simulink model "eeg_sim"  (R2025b)
settings: Solver=VariableStepAuto  StartTime=0.0  StopTime=10000  RelTol=1e-3
libraries: dspnetwork x1
settings Model: Creator=rashe  LastModifiedBy=rashe

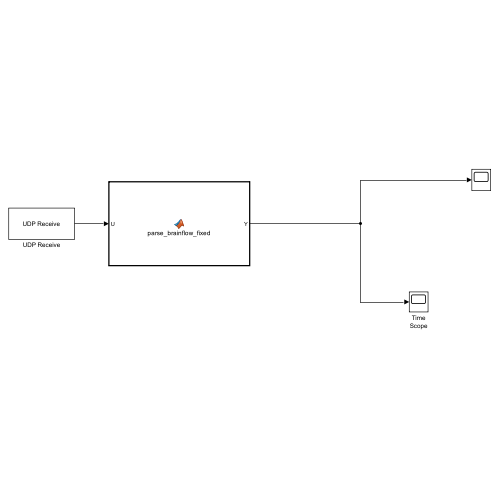
[thumbnail: Simulink's stored preview of the top-level diagram]
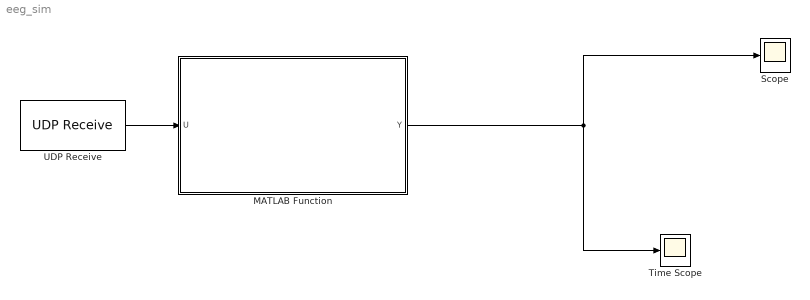
== system eeg_sim ==
  MATLAB Function : MATLAB Function  TreatAsAtomicUnit=on
  Scope : Scope
      settings: ActiveDisplayYMinimum=-2.2008671227142039E+8  ActiveDisplayYMaximum=1.9807758069769027E+9
  Time Scope : Scope
      settings: TimeUnits=Metric (based on Time Span)  YLabel=Amplitude
  UDP Receive : dspnetwork/UDP Receive  localURL='0.0.0.0'  localPort=25000  remoteURL='0.0.0.0'  remotePort=-1  recvBufferSize=65535  dims=65507  signalDatatype=uint8  isComplex=off  isVarSize=on  showBlockingTime=off  blockingTime=0  sampletime=0.004  blockPlatform=[]
      settings: LibrarySourceBlock=dspsrcs4/UDP Receive
  wires:
  UDP Receive/1 -> MATLAB Function/1(U)
  MATLAB Function/1(Y) -> Time Scope/1, Scope/1

== matlab function eeg_sim/MATLAB Function ==
  data: U input; Y output
function Y = parse_brainflow_fixed(U)
%#codegen
NumRows  = int32(13);
KeepRows = int32([2 3 4 5 6 7 8 9 12]);
FrameCols = 1;                        % choose your frame width

nKeep = numel(KeepRows);
coder.varsize('buf',[13,FrameCols],[false false]);

% persistent buffer of doubles
persistent buf nfill
if isempty(nfill), buf = zeros(double(NumRows), FrameCols); nfill = 0; end

% Default output (fixed size)
Y = nan(nKeep, FrameCols);

if ~isempty(U)
    d = typecast(uint8(U(:)),'double');
    cols = floor(numel(d)/double(NumRows));
    if cols > 0
        D = reshape(d(1:cols*double(NumRows)), double(NumRows), cols);
        take = min(cols, FrameCols - nfill);
        buf(:, nfill+1:nfill+take) = D(:,1:take);
        nfill = nfill + take;
    end
end

if nfill < FrameCols
    % not enough new data yet -> output current buffer (partially filled with old/NaN)
    Y = buf(double(KeepRows), :);
else
    Y = buf(double(KeepRows), :);
    nfill = 0;   % reset buffer
end
